simulink model "Marine_LocoMotive_UAV"  (R2018a)
settings: Solver=ode4  StartTime=0.0  StopTime=80  FixedStep=T  RelTol=1e-3
values from neighbouring files (symbols this model uses):
  a_11 = 0.05*m_b    (= 0.625)    [Marine_LocoMotive_UAV.m]
  a_33 = m_b    (= 12.5)    [Marine_LocoMotive_UAV.m]
  A_w = 1*1.5/2    (= 0.75)    [Marine_LocoMotive_UAV.m]
  A_w2 = 1*0.27/2    (= 0.135)    [Marine_LocoMotive_UAV.m]
  Ac = 0.0331    [Marine_LocoMotive_UAV.m]
  alpha_bar = pi/4    (= 0.785398163397)    [Marine_LocoMotive_UAV.m]
  Am = sysd.denominator{1}    [Marine_LocoMotive_UAV.m]
  Am1_LPF = sysd.denominator{1}    [Marine_LocoMotive_UAV.m]
  Am2_LPF = sysd.denominator{1}    [Marine_LocoMotive_UAV.m]
  Am_asw_LPF = sysd.denominator{1}    [Marine_LocoMotive_UAV.m]
  Am_coup_LPF = sysd.denominator{1}    [Marine_LocoMotive_UAV.m]
  Am_rdeL_LPF = sysd.denominator{1}    [Marine_LocoMotive_UAV.m]
  Am_reL_LPF = sysd.denominator{1}    [Marine_LocoMotive_UAV.m]
  Am_rref20_LPF = sysd.denominator{1}    [Marine_LocoMotive_UAV.m]
  Am_rref_LPF = sysd.denominator{1}    [Marine_LocoMotive_UAV.m]
  AmAlpha_LPF = sysd.denominator{1}    [Marine_LocoMotive_UAV.m]
  Amp_sf = 3    [Marine_LocoMotive_UAV.m]
  AmV_LPF = sysd.denominator{1}    [Marine_LocoMotive_UAV.m]
  AmZ_LPF = sysd.denominator{1}    [Marine_LocoMotive_UAV.m]
  b_11 = 0    [Marine_LocoMotive_UAV.m]
  b_33 = 2*m_b*omega_h    (= 27.5578302946)    [Marine_LocoMotive_UAV.m]
  Bm = sysd.numerator{1}    [Marine_LocoMotive_UAV.m]
  Bm1_LPF = sysd.numerator{1}    [Marine_LocoMotive_UAV.m]
  Bm2_LPF = sysd.numerator{1}    [Marine_LocoMotive_UAV.m]
  Bm_asw_LPF = sysd.numerator{1}    [Marine_LocoMotive_UAV.m]
  Bm_coup_LPF = sysd.numerator{1}    [Marine_LocoMotive_UAV.m]
  Bm_rdeL_LPF = sysd.numerator{1}    [Marine_LocoMotive_UAV.m]
  Bm_reL_LPF = sysd.numerator{1}    [Marine_LocoMotive_UAV.m]
  Bm_rref20_LPF = sysd.numerator{1}    [Marine_LocoMotive_UAV.m]
  Bm_rref_LPF = sysd.numerator{1}    [Marine_LocoMotive_UAV.m]
  BmAlpha_LPF = sysd.numerator{1}    [Marine_LocoMotive_UAV.m]
  BmV_LPF = sysd.numerator{1}    [Marine_LocoMotive_UAV.m]
  BmZ_LPF = sysd.numerator{1}    [Marine_LocoMotive_UAV.m]
  C_S = [5;9]*10^-3    [Marine_LocoMotive_UAV.m]
  Cd_u = 0.2    [Marine_LocoMotive_UAV.m]
  D_x = b_11 + D_s(1)    [Marine_LocoMotive_UAV.m]
  D_z = b_33 + D_s(2)    [Marine_LocoMotive_UAV.m]
  dc_M_p = 6.7    [Marine_LocoMotive_UAV.m]
  Delta_h = (A_im/A_b-0.5)*h_b    (= -0.0625)    [Marine_LocoMotive_UAV.m]
  eps_V = 0.1    [Marine_LocoMotive_UAV.m]
  epsilon_1 = 5    [Marine_LocoMotive_UAV.m]
  epsilon_e_u1 = 0.05    [Marine_LocoMotive_UAV.m]
  epsilon_w = 0    [Marine_LocoMotive_UAV.m]
  epsilon_w2 = pi    (= 3.14159265359)    [Marine_LocoMotive_UAV.m]
  g = 9.81    [Marine_LocoMotive_UAV.m]
  gamma_d_p = (2*0.3/0.03*2*0.2*12/4)/10    (= 2.4)    [Marine_LocoMotive_UAV.m]
  H = 10    [Marine_LocoMotive_UAV.m]
  h_b = 0.25    [Marine_LocoMotive_UAV.m]
  J_b = m_b*h_b*l_b/12    (= 0.208333333333)    [Marine_LocoMotive_UAV.m]
  J_u = 0.03    [Marine_LocoMotive_UAV.m]
  K = 40    [Marine_LocoMotive_UAV.m]
  k3 = 24    [Marine_LocoMotive_UAV.m]
  k4 = 0.8    [Marine_LocoMotive_UAV.m]
  k_w = omega_w^2/g    (= 0.123862835563)    [Marine_LocoMotive_UAV.m]
  k_w2 = omega_w2^2/g    (= 0.447144836384)    [Marine_LocoMotive_UAV.m]
  kd_a = 5.6    [Marine_LocoMotive_UAV.m]
  kd_r = 19.5    [Marine_LocoMotive_UAV.m]
  kd_t = 10    [Marine_LocoMotive_UAV.m]
  kd_x = 5    [Marine_LocoMotive_UAV.m]
  kd_z = 2    [Marine_LocoMotive_UAV.m]
  ki_a = 1.6    [Marine_LocoMotive_UAV.m]
  ki_r = 9    [Marine_LocoMotive_UAV.m]
  ki_T = 12    [Marine_LocoMotive_UAV.m]
  ki_x = 1.2    [Marine_LocoMotive_UAV.m]
  ki_z = 1    [Marine_LocoMotive_UAV.m]
  kp_a = 9.6    [Marine_LocoMotive_UAV.m]
  kp_r = 45    [Marine_LocoMotive_UAV.m]
  kp_t = 20    [Marine_LocoMotive_UAV.m]
  kp_T = 25    [Marine_LocoMotive_UAV.m]
  kp_x = 7    [Marine_LocoMotive_UAV.m]
  kp_z = 3    [Marine_LocoMotive_UAV.m]
  L = 0.2    [Marine_LocoMotive_UAV.m]
  l_b = 0.8    [Marine_LocoMotive_UAV.m]
  Lc_0 = 7    [Marine_LocoMotive_UAV.m]
  LIMIT_CMD_PITCH = 45*pi/180    (= 0.785398163397)    [Marine_LocoMotive_UAV.m]
  LIMIT_uCMD_HEIGHT = 3.5*K    (= 140)    [Marine_LocoMotive_UAV.m]
  m_b = rho_w*Vol_b/4    (= 12.5)    [Marine_LocoMotive_UAV.m]
  m_u = 1.8    [Marine_LocoMotive_UAV.m]
  min_sf = 5    [Marine_LocoMotive_UAV.m]
  nu_w = 1.787*10^-6    (= 1.787e-06)    [Marine_LocoMotive_UAV.m]
  omega_w = 2*pi/T_w    (= 1.10231321179)    [Marine_LocoMotive_UAV.m]
  omega_w2 = 2*pi/T_w2    (= 2.09439510239)    [Marine_LocoMotive_UAV.m]
  r_0 = sqrt( (X0_b(1) - X0_u(1))^2 +(X0_b(2) - X0_u(2))^2 )    [Marine_LocoMotive_UAV.m]
  r_bar = Lc_0-0.3    (= 6.7)    [Marine_LocoMotive_UAV.m]
  r_min = (zu_bar-H)-0.2    [Marine_LocoMotive_UAV.m]
  rho_a = 1.225    [Marine_LocoMotive_UAV.m]
  rho_w = 1000    [Marine_LocoMotive_UAV.m]
  T = 1/500    (= 0.002)    [Marine_LocoMotive_UAV.m]
  T_init = 10    [Marine_LocoMotive_UAV.m]
  Theta0 = 0*atan2(V_bar*D_x*cos(alpha_bar_0),V_bar*D_x*sin(alpha_bar_0)+m_u*g*cos(alpha_bar_0))    [Marine_LocoMotive_UAV.m]
  u_s = w_dir*A_w^2*omega_w*k_w*exp(2*k_w*(-Delta_h/2))    [Marine_LocoMotive_UAV.m]
  u_s2 = w_dir2*A_w2^2*omega_w2*k_w2*exp(2*k_w2*(-Delta_h/2))    [Marine_LocoMotive_UAV.m]
  u_t = -1*0.5*1    (= -0.5)    [Marine_LocoMotive_UAV.m]
  u_w = 0*0.2    (= 0)    [Marine_LocoMotive_UAV.m]
  V0_b = [u_t+u_w+u_s+v_x_w, v_z_w]    [Marine_LocoMotive_UAV.m]
  V0_u = [0 0]    [Marine_LocoMotive_UAV.m]
  V_bar = 4    [Marine_LocoMotive_UAV.m]
  Vol_b = A_b*l_b    (= 0.05)    [Marine_LocoMotive_UAV.m]
  w_dir = 1    [Marine_LocoMotive_UAV.m]
  w_dir2 = 1    [Marine_LocoMotive_UAV.m]
  X0_b = [0,H-Delta_h]    [Marine_LocoMotive_UAV.m]
  X0_u = X0_b + [3 3]    [Marine_LocoMotive_UAV.m]
  zu_bar = X0_b(2) + Lc_0*sin(alpha_bar_0)    [Marine_LocoMotive_UAV.m]
undefined symbols (not defined in the file or in its folder): Am_HPF, Am_LPF, Am_LPF2, an1, an1_v, an2, an3, Bm_HPF, Bm_LPF, Bm_LPF2, bn1, bn1_v, bn2, bn3, DiscIntNeverNeededParam, F, Light, magnitude, MIL, OMEGA_FILTER_OUTER, R_b, Tc, Tg, Tn, Ts, Tsc, Tz, X_GPS_offset
libraries: simulink x50, simulink_extras x9, aerolibwind2 x2
(part 3 of 6)

== system Marine_LocoMotive_UAV/Sensors and Filters/Sensors ==
  note: Gyro noise destroys the estimation
  note: Acc noise does not affect estimation
  "q " : Inport
  Ab : Inport  Port=2
  Xe : Inport  Port=3
  Euler : Inport  Port=4
  " Sonar (10Hz) (true elevation instead real sonar signal)" : Subsystem
  Accelerometer (500Hz) : Subsystem  TreatAsAtomicUnit=on  SystemSampleTime=Ts
  "GPS (10Hz) " : Subsystem  TreatAsAtomicUnit=on  SystemSampleTime=Tg
  Gyro (500Hz) : Subsystem  TreatAsAtomicUnit=on  SystemSampleTime=Ts
  RT : RateTransition  OutPortSampleTime=Ts
  Rate Transition : RateTransition
  Rate Transition1 : RateTransition
  Rate Transition2 : RateTransition  Deterministic=off  InitialCondition=[X0_u Theta0 1 1]
  Z : Selector  InputPortWidth=5  IndexOptions=Index vector (dialog)  Indices=2  OutputSizes=1
  acc : Scope  Commented=on
  pqr : Scope  Commented=on
  rotation matrix R : Subsystem
  Acc : Outport
  GPS : Outport  Port=2
  " q" : Outport  Port=3
  Sonar : Outport  Port=4
  wires:
  Xe/1 -> "GPS (10Hz) "/1(Xe)
  Ab/1 -> RT/1
  "q "/1 -> Gyro (500Hz)/1(q)
  Euler/1 -> rotation matrix R/1(angle (rad)), "GPS (10Hz) "/2(Euler)
  Accelerometer (500Hz)/1(Acc) -> Rate Transition1/1
  Gyro (500Hz)/1(" q") -> Rate Transition/1
  Z/1 -> " Sonar (10Hz) (true elevation instead real sonar signal)"/1(sonar (m))
  " Sonar (10Hz) (true elevation instead real sonar signal)"/1(calib sonar (m)) -> Sonar/1
  Rate Transition/1 -> pqr/1, " q"/1
  Rate Transition1/1 -> acc/1, Acc/1
  RT/1 -> Accelerometer (500Hz)/1(Ab)
  rotation matrix R/1(R) -> "GPS (10Hz) "/3(DCM_b2e)
  Rate Transition2/1 -> Z/1, GPS/1
  "GPS (10Hz) "/1(GPS) -> Rate Transition2/1

== system Marine_LocoMotive_UAV/Sensors and Filters/Sterio camera + encoder ==
  note: the error in alpha should relate to the stereo camera accuracy and the radial distance:
      | alpha = atan( 2cm / 7 m) = 0.0029 rad.
  alpha : Inport
  alpha_dot : Inport  Port=2
  alpha_ddot : Inport  Port=3
  r : Inport  Port=4
  r_dot : Inport  Port=5
  r_ddot : Inport  Port=6
  Discrete Derivative{,1..3} (4 alike) : simulink/Discrete/Discrete Derivative  gainval=1.0  ICPrevScaledInput=0.0  OutMin=[]  OutMax=[]  OutDataType=fixdt(1, 16)  OutScaling=2^-10  DoSatur=off
  Gain1 : Gain  Gain=0.5
  Gain2 : Gain  Gain=0.3
  Gain4 : Gain
  Gain5 : Gain
  Gain6 : Gain  Gain=0.25
  Gain7 : Gain  Gain=0.5
  Low Pass Filter{1..9} (9 alike) : DiscreteTransferFcn  Numerator=Bm_LPF2  Denominator=Am_LPF2
  Low Pass Filter10 : DiscreteTransferFcn  Commented=on  Numerator=Bm_LPF2  Denominator=Am_LPF2
  Low Pass Filter11 : DiscreteTransferFcn  Commented=on  Numerator=Bm_LPF2  Denominator=Am_LPF2
  Rate Transition1 : RateTransition
  Rate Transition2 : RateTransition
  Sum{1..2,7..10} (6 alike) : Sum  Inputs=++|
  stereo cam noise (location in frame) : RandomNumber  Variance=1/100000  Seed=5684  SampleTime=Tsc
  sterio cam noise (range) : RandomNumber  Variance=1/1000  Seed=1142  SampleTime=Tsc
  alpha_est : Outport
  alpha_dot_est : Outport  Port=2
  r_est : Outport  Port=3
  r_dot_est : Outport  Port=4
  alpha_ddot_est : Outport  Port=5
  r_ddot_est : Outport  Port=6
  wires:
  Rate Transition2/1 -> Low Pass Filter3/1
  stereo cam noise (location in frame)/1 -> Rate Transition2/1
  Gain5/1 -> Sum8/1
  Sum10/1 -> r_dot_est/1
  Discrete Derivative/1 -> Low Pass Filter8/1
  alpha_dot/1 -> Sum9/2
  Gain4/1 -> Sum7/1
  Discrete Derivative1/1 -> Low Pass Filter7/1
  Sum7/1 -> alpha_est/1
  Sum8/1 -> r_est/1
  r/1 -> Sum8/2
  alpha/1 -> Sum7/2
  r_dot/1 -> Sum10/2
  Sum9/1 -> alpha_dot_est/1
  sterio cam noise (range)/1 -> Rate Transition1/1
  Rate Transition1/1 -> Low Pass Filter1/1
  Sum1/1 -> alpha_ddot_est/1
  Discrete Derivative2/1 -> Low Pass Filter6/1
  Gain6/1 -> Discrete Derivative2/1, Sum9/1
  Gain1/1 -> Sum1/1
  alpha_ddot/1 -> Sum1/2
  r_ddot/1 -> Sum2/2
  Discrete Derivative3/1 -> Low Pass Filter9/1
  Gain2/1 -> Sum2/1
  Sum2/1 -> r_ddot_est/1
  Gain7/1 -> Discrete Derivative3/1, Sum10/1
  Low Pass Filter2/1 -> Gain7/1
  Low Pass Filter4/1 -> Gain2/1
  Low Pass Filter5/1 -> Gain6/1
  Low Pass Filter6/1 -> Gain1/1
  Low Pass Filter7/1 -> Low Pass Filter5/1
  Low Pass Filter8/1 -> Low Pass Filter2/1
  Low Pass Filter9/1 -> Low Pass Filter4/1
  Low Pass Filter3/1 -> Gain4/1, Discrete Derivative1/1
  Low Pass Filter1/1 -> Gain5/1, Discrete Derivative/1

== system Marine_LocoMotive_UAV/Sensors and Filters/quadrotor position from relative buoy-UAV position ==
  X_u : Inport
  Xdot_u : Inport  Port=2
  Xddot_u : Inport  Port=3
  r : Inport  Port=4
  r_dot : Inport  Port=5
  r_ddot : Inport  Port=6
  alpha : Inport  Port=7
  alpha_dot : Inport  Port=8
  alpha_ddot : Inport  Port=9
  Demux : Demux  Outputs=2
  Gain1 : Gain  Gain=-1
  Gain2 : Gain  Gain=2
  Product1 : Product  Inputs=3
  Product{2,4..5,7..8} (5 alike) : Product
  Product3 : Product  Multiplication=Matrix(*)
  Product6 : Product  Multiplication=Matrix(*)
  Sum : Sum  Inputs=|+-
  Sum1 : Sum  Inputs=|+-
  Sum2 : Sum  Inputs=+-|
  Sum3 : Sum  Inputs=++|
  Sum4 : Sum  Inputs=+-|
  Trigonometric Function : Trigonometry  Operator=sincos
  Vector Concatenate{1..4} (4 alike) : Concatenate
  r1 : InportShadow  Port=4
  r_dot1 : InportShadow  Port=5
  "rotation matrix R " : Subsystem
  theta u{1..2,4,6} (4 alike) : Scope
  Xb : Outport
  Xdot_b : Outport  Port=2
  Xddot_b : Outport  Port=3
  wires:
  Trigonometric Function/2 -> Product5/1
  Trigonometric Function/1 -> Product4/1
  alpha/1 -> "rotation matrix R "/1(angle (rad)), Trigonometric Function/1  "alpha"
  Sum1/1 -> Vector Concatenate3/2
  Vector Concatenate3/1 -> theta u4/1, Xb/1
  Product5/1 -> Sum/2
  Demux/2 -> Sum1/1  "z_u"
  Product4/1 -> Sum1/2
  Sum/1 -> Vector Concatenate3/1
  X_u/1 -> Demux/1
  Demux/1 -> Sum/1  "x_u"
  Vector Concatenate2/1 -> Product3/2
  Sum4/1 -> Xdot_b/1, theta u6/1
  Product3/1 -> Sum4/2
  r/1 -> Product2/1, Product5/2, Product4/2
  r_dot/1 -> theta u1/1, Vector Concatenate2/1
  Product2/1 -> theta u2/1, Vector Concatenate2/2
  alpha_dot/1 -> Product2/2, Product7/1, Product1/2, Product1/1
  Xdot_u/1 -> Sum4/1
  Product6/1 -> Sum2/2
  Gain2/1 -> Vector Concatenate1/2
  "rotation matrix R "/1(R) -> Product6/1, Product3/1
  Product1/1 -> Gain1/1
  Sum3/1 -> Product6/2
  r1/1 -> Product8/1, Product1/3
  Product7/1 -> Gain2/1
  r_dot1/1 -> Product7/2
  Xddot_u/1 -> Sum2/1
  Vector Concatenate1/1 -> Sum3/2
  r_ddot/1 -> Vector Concatenate4/1
  Product8/1 -> Vector Concatenate4/2
  alpha_ddot/1 -> Product8/2
  Vector Concatenate4/1 -> Sum3/1
  Gain1/1 -> Vector Concatenate1/1
  Sum2/1 -> Xddot_b/1

== system Marine_LocoMotive_UAV/UAV controller/Coupling ==
  U1 : Inport
  U3 : Inport  Port=2
  Coupling : Subsystem
  sat : Subsystem
  u_1 : Outport
  theta_d : Outport  Port=2
  wires:
  Coupling/1(u1 (N)) -> u_1/1
  Coupling/2(phi_d (rad)) -> sat/1(u)
  U3/1 -> Coupling/2(U3)
  U1/1 -> Coupling/1(U1)
  sat/1(sat(u)) -> theta_d/1

== system Marine_LocoMotive_UAV/UAV controller/Coupling  ==
  u_T : Inport
  u_a : Inport  Port=2
  alpha : Inport  Port=3
  Add5 : Sum  Inputs=2
  Bias : Bias  Bias=-pi/2
  Product1 : Product
  Product3 : Product
  Saturation : Saturate  UpperLimit=LIMIT_uCMD_HEIGHT  LowerLimit=m_u*g*0.5
  Scope{,1..5} (6 alike) : Scope
  Sqrt : Sqrt  SaturateOnIntegerOverflow=on
  Subtract : Sum  Inputs=--
  Trigonometric Function1 : Trigonometry  Operator=atan2
  Vector Concatenate : Concatenate
  "sat " : Subsystem
  u1 : Outport
  theta_c : Outport  Port=2
  wires:
  Bias/1 -> Scope2/1, Subtract/1
  Product1/1 -> Add5/1, Scope/1
  Sqrt/1 -> Saturation/1
  Subtract/1 -> "sat "/1(u)
  Trigonometric Function1/1 -> Scope4/1, Subtract/2
  Product3/1 -> Scope1/1, Add5/2
  Add5/1 -> Sqrt/1
  alpha/1 -> Bias/1
  Saturation/1 -> u1/1
  "sat "/1(sat(u)) -> Scope3/1, theta_c/1
  u_a/1 -> Vector Concatenate/1, Trigonometric Function1/1, Product3/1, Product3/2
  u_T/1 -> Product1/2, Product1/1, Vector Concatenate/2, Trigonometric Function1/2
  Vector Concatenate/1 -> Scope5/1

== system Marine_LocoMotive_UAV/UAV controller/Enabled Subsystem1 ==
  u : Inport
  reset : Inport  Port=2
  u0 : Inport  Port=3
  Enable : EnablePort
  Logical Operator : Logic  Operator=NOT  AllPortsSameDT=off  OutDataTypeStr=boolean
  Low Pass Filter5 : DiscreteTransferFcn  Numerator=Bm_rdeL_LPF  Denominator=Am_rdeL_LPF  InitialStatesSource=Input port  ExternalReset=Level
      settings: InputPortMap=u0,r7,p5
  Mux2 : Mux  Inputs=2
  adjustment for this specific transfer function : Gain  Gain=84.6505602
  r_dot filt : Scope
  r_dot filt1 : Scope
  y : Outport
  wires:
  u/1 -> Mux2/2, Low Pass Filter5/1
  Low Pass Filter5/1 -> Mux2/1, y/1
  Logical Operator/1 -> r_dot filt1/1, Low Pass Filter5/2
  u0/1 -> adjustment for this specific transfer function/1
  Mux2/1 -> r_dot filt/1
  adjustment for this specific transfer function/1 -> Low Pass Filter5/3
  reset/1 -> Logical Operator/1

== system Marine_LocoMotive_UAV/UAV controller/V controller ==
  V_bar : Inport
  V : Inport  Port=2
  Discrete Derivative1 : simulink/Discrete/Discrete Derivative  gainval=1.0  ICPrevScaledInput=0.0  OutMin=[]  OutMax=[]  OutDataType=fixdt(1, 16)  OutScaling=2^-10  DoSatur=off
  Discrete Derivative6 : simulink/Discrete/Discrete Derivative  gainval=1.0  ICPrevScaledInput=0.0  OutMin=[]  OutMax=[]  OutDataType=fixdt(1, 16)  OutScaling=2^-10  DoSatur=off
  Discrete-Time Integrator : DiscreteIntegrator  SampleTime=-1  LimitOutput=on  UpperSaturationLimit=300  LowerSaturationLimit=-200  ICPrevOutput=DiscIntNeverNeededParam  ICPrevScaledInput=DiscIntNeverNeededParam
  Gain : Gain  Gain=ki_x
  IC : InitialCondition  Value=0
  IC1 : InitialCondition  Value=0
  IC2 : InitialCondition  Value=0
  K1 : Gain  Gain=kp_x
  K2 : Gain  Gain=kd_x
  K3 : Gain
  K4 : Gain
  Mux : Mux  Inputs=2
  Mux1 : Mux  Inputs=2
  Product : Product
  Saturation1 : Saturate  UpperLimit=50  LowerLimit=-20
  Scope{1..6} (6 alike) : Scope
  Step : Step  Time=3*T  SampleTime=0
  Sum : Sum  Inputs=|+-
  Sum1 : Sum  Inputs=|+-
  Sum4 : Sum  Inputs=---
  U1 (m/s^2) : Outport
  wires:
  Sum1/1 -> Product/1  "ev"
  Sum/1 -> Discrete-Time Integrator/1, K1/1  "ex"
  V_bar/1 -> Mux/2, Sum/2, Discrete Derivative6/1
  Sum4/1 -> Saturation1/1
  K1/1 -> K4/1
  K2/1 -> K3/1
  Discrete-Time Integrator/1 -> Gain/1
  Gain/1 -> Scope3/1, Sum4/3
  Saturation1/1 -> Scope4/1, U1 (m/s^2)/1
  Mux/1 -> Scope1/1
  Discrete Derivative1/1 -> IC1/1
  Mux1/1 -> Scope2/1
  Discrete Derivative6/1 -> IC2/1
  IC/1 -> Discrete Derivative1/1, Mux/1, Sum/1
  V/1 -> IC/1
  IC1/1 -> Sum1/1, Mux1/1
  IC2/1 -> Mux1/2, Sum1/2
  K3/1 -> Scope5/1, Sum4/2
  K4/1 -> Scope6/1, Sum4/1
  Product/1 -> K2/1
  Step/1 -> Product/2

== system Marine_LocoMotive_UAV/UAV controller/Z controller ==
  z_bar : Inport
  z_u : Inport  Port=2
  Constant : Constant  Value=g
  Discrete Derivative1 : simulink/Discrete/Discrete Derivative  gainval=1.0  ICPrevScaledInput=0.0  OutMin=[]  OutMax=[]  OutDataType=fixdt(1, 16)  OutScaling=2^-10  DoSatur=off
  Discrete Derivative6 : simulink/Discrete/Discrete Derivative  gainval=1.0  ICPrevScaledInput=0.0  OutMin=[]  OutMax=[]  OutDataType=fixdt(1, 16)  OutScaling=2^-10  DoSatur=off
  Discrete-Time Integrator : DiscreteIntegrator  SampleTime=-1  LimitOutput=on  UpperSaturationLimit=100  LowerSaturationLimit=-100  ICPrevOutput=DiscIntNeverNeededParam  ICPrevScaledInput=DiscIntNeverNeededParam
  Divide : Product  Inputs=*/
  Gain : Gain  Gain=ki_z
  IC : InitialCondition  Value=0
  IC1 : InitialCondition  Value=0
  K1 : Gain  Gain=kp_z
  K2 : Gain  Gain=kd_z
  K3 : Gain
  Mux : Mux  Inputs=2
  Mux1 : Mux  Inputs=2
  Saturation1 : Saturate  UpperLimit=inf  LowerLimit=g/2
  Scope{1..6} (6 alike) : Scope
  Sum : Sum  Inputs=|+-
  Sum1 : Sum  Inputs=|+-
  Sum2 : Sum  Inputs=|++
  Sum4 : Sum  Inputs=---
  Trigonometric Function : Trigonometry  Operator=cos
  U3 (m/s^2) : Outport
  wires:
  Gain/1 -> Scope3/1, Sum4/3
  Discrete-Time Integrator/1 -> Gain/1
  K2/1 -> Scope5/1, Sum4/2
  K1/1 -> K3/1
  Sum4/1 -> Sum2/1
  Discrete Derivative1/1 -> IC/1
  Discrete Derivative6/1 -> IC1/1
  z_u/1 -> Discrete Derivative1/1, Mux/1, Sum/1
  Sum/1 -> K1/1, Discrete-Time Integrator/1  "ex"
  Sum1/1 -> K2/1  "ev"
  z_bar/1 -> Mux/2, Sum/2, Discrete Derivative6/1
  Mux/1 -> Scope1/1
  Mux1/1 -> Scope2/1
  Saturation1/1 -> U3 (m/s^2)/1, Scope4/1
  IC/1 -> Mux1/1, Sum1/1
  IC1/1 -> Mux1/2, Sum1/2
  K3/1 -> Scope6/1, Sum4/1
  [theta_u] -> Trigonometric Function/1
  Trigonometric Function/1 -> Divide/2
  Sum2/1 -> Saturation1/1
  Constant/1 -> Divide/1
  Divide/1 -> Sum2/2

== system Marine_LocoMotive_UAV/UAV controller/cond1 ==
  r : Inport
  r_dot : Inport  Port=2
  coupled : Inport  Port=3
  Constant : Constant  Value=Lc_0
  Constant2 : Constant  Value=T
  MATLAB Function : MATLAB Function  TreatAsAtomicUnit=on
  r_dot filt2 : Scope
  key : Outport
  wires:
  r/1 -> MATLAB Function/1(r)
  Constant/1 -> MATLAB Function/4(Lc)
  Constant2/1 -> MATLAB Function/5(dt)
  MATLAB Function/1(y) -> key/1
  r_dot/1 -> MATLAB Function/2(r_dot)
  coupled/1 -> MATLAB Function/3(coupled)
  MATLAB Function/2(t) -> r_dot filt2/1

== system Marine_LocoMotive_UAV/UAV controller/pitch control ==
  theta_d : Inport
  theta_q : Inport  Port=2
  omega_q : Inport  Port=3
  Constant : Constant  Value=J_u
  Discrete Transfer Fcn : DiscreteTransferFcn  Numerator=Bm1_LPF  Denominator=Am1_LPF
  Discrete Transfer Fcn1 : DiscreteTransferFcn  Numerator=Bm2_LPF  Denominator=Am2_LPF
  Discrete Derivative3 : simulink/Discrete/Discrete Derivative  gainval=1.0  ICPrevScaledInput=Theta0/T  OutMin=[]  OutMax=[]  OutDataType=fixdt(1, 16)  OutScaling=2^-10  DoSatur=off
  Discrete Derivative4 : simulink/Discrete/Discrete Derivative  gainval=1.0  ICPrevScaledInput=0.0  OutMin=[]  OutMax=[]  OutDataType=fixdt(1, 16)  OutScaling=2^-10  DoSatur=off
  Discrete Derivative6 : simulink/Discrete/Discrete Derivative  gainval=1.0  ICPrevScaledInput=Theta0/T  OutMin=[]  OutMax=[]  OutDataType=fixdt(1, 16)  OutScaling=2^-10  DoSatur=off
  Discrete-Time Integrator : DiscreteIntegrator  SampleTime=-1  LimitOutput=on  UpperSaturationLimit=dc_M_p  LowerSaturationLimit=-dc_M_p  ICPrevOutput=DiscIntNeverNeededParam  ICPrevScaledInput=DiscIntNeverNeededParam
  Gain : Gain  Gain=gamma_d_p
  IC : InitialCondition  Value=0
  IC2 : InitialCondition  Value=0
  Integrator : Integrator  Commented=on  LimitOutput=on  UpperSaturationLimit=dc_M_p  LowerSaturationLimit=-dc_M_p
  K1 : Gain  Gain=kp_t
  K2 : Gain  Gain=kd_t
  K3 : Gain  Gain=1+k3*k4
  K4 : Gain  Gain=k3+k4
  K5 : Gain
  K6 : Gain
  Mux : Mux  Inputs=2
  Mux1 : Mux  Inputs=3
  Mux2 : Mux  Inputs=2
  Product1 : Product
  Saturation : Saturate  UpperLimit=[5]  LowerLimit=[-5]
  Saturation - Limit Height Controller1 : Saturate  UpperLimit=K*L*1.41/4  LowerLimit=-K*L*1.41/4
  Saturation - Limit Height Controller2 : Saturate  UpperLimit=15  LowerLimit=-15
  Sum : Sum  Inputs=|+-
  Sum1 : Sum  Inputs=|+-
  Sum4 : Sum  Inputs=--+-
  T2 {,1..9} (10 alike) : Scope
  theta_d1 : InportShadow
  M1 (N.m) : Outport
  wires:
  Product1/1 -> Saturation - Limit Height Controller1/1
  Saturation - Limit Height Controller1/1 -> "T2 "/1, M1 (N.m)/1
  Sum1/1 -> K2/1  "ev"
  Sum4/1 -> Product1/1
  Discrete Derivative6/1 -> IC/1
  Discrete Derivative3/1 -> IC2/1
  Discrete Transfer Fcn1/1 -> Mux2/1, Saturation/1
  Sum/1 -> K1/1, Discrete-Time Integrator/1  "ex"
  K1/1 -> T2 7/1, Sum4/1
  K2/1 -> K6/1
  Discrete-Time Integrator/1 -> Gain/1
  Gain/1 -> K5/1, T2 5/1
  Constant/1 -> Product1/2
  Mux/1 -> T2 1/1
  theta_q/1 -> Mux/1, Sum/1
  omega_q/1 -> Mux1/1, Sum1/1
  Mux1/1 -> T2 2/1
  Discrete Transfer Fcn/1 -> Mux1/2, Sum1/2  "ex"
  Discrete Derivative4/1 -> Mux2/2, Discrete Transfer Fcn1/1, T2 3/1
  theta_d/1 -> Mux/2, Sum/2, Discrete Derivative6/1
  Saturation/1 -> T2 8/1, Sum4/3
  IC/1 -> Mux1/3, Discrete Transfer Fcn/1
  theta_d1/1 -> Discrete Derivative3/1
  IC2/1 -> Discrete Derivative4/1
  K5/1 -> Sum4/4
  Mux2/1 -> T2 4/1
  K6/1 -> T2 6/1, Sum4/2

== system Marine_LocoMotive_UAV/UAV controller/rdot 0 ==
  X : Inport
  Trigger : TriggerPort  VariantControl=Variant
  Xu_init : Outport
  wires:
  X/1 -> Xu_init/1

== system Marine_LocoMotive_UAV/UAV controller/switch controllers ==
  radial position : Inport
  buoy velocity : Inport  Port=2
  coupled : Inport  Port=3
  active : Inport  Port=4
  r : Inport  Port=5
  Abs1 : Abs  Commented=on
  Compare To Constant : simulink/Logic and Bit Operations/Compare To Constant  relop=>=  const=Lc_0-0.1  OutDataTypeStr=boolean
  Compare To Constant1 : simulink/Logic and Bit Operations/Compare To Constant  Commented=on  relop=<=  const=0.3  OutDataTypeStr=boolean
  Logical Operator1 : Logic  AllPortsSameDT=off  OutDataTypeStr=boolean
  Logical Operator2 : Logic  Operator=OR  AllPortsSameDT=off  OutDataTypeStr=boolean
  Mux1 : Mux  Inputs=2
  Mux2 : Mux  Inputs=2
  Smooth channel switching : Subsystem  Commented=on
  Switch : Switch  Criteria=u2 > Threshold
  smooth switch : Subsystem
  u_T1 : Scope
  u_T2 : Scope
  u_T3 : Scope
  u_T : Outport
  wires:
  buoy velocity/1 -> smooth switch/2(u 2), Switch/1, Mux2/2
  Logical Operator1/1 -> u_T2/1, smooth switch/3(switch), Switch/2
  coupled/1 -> Logical Operator2/2
  radial position/1 -> smooth switch/1(u 1), Switch/3, Mux2/1
  Switch/1 -> Mux1/1
  Mux2/1 -> u_T1/1
  active/1 -> Logical Operator1/2
  Logical Operator2/1 -> Logical Operator1/1
  r/1 -> Compare To Constant/1
  Compare To Constant/1 -> Logical Operator2/1
  Abs1/1 -> Compare To Constant1/1
  Mux1/1 -> u_T3/1
  smooth switch/1(y) -> u_T/1, Mux1/2

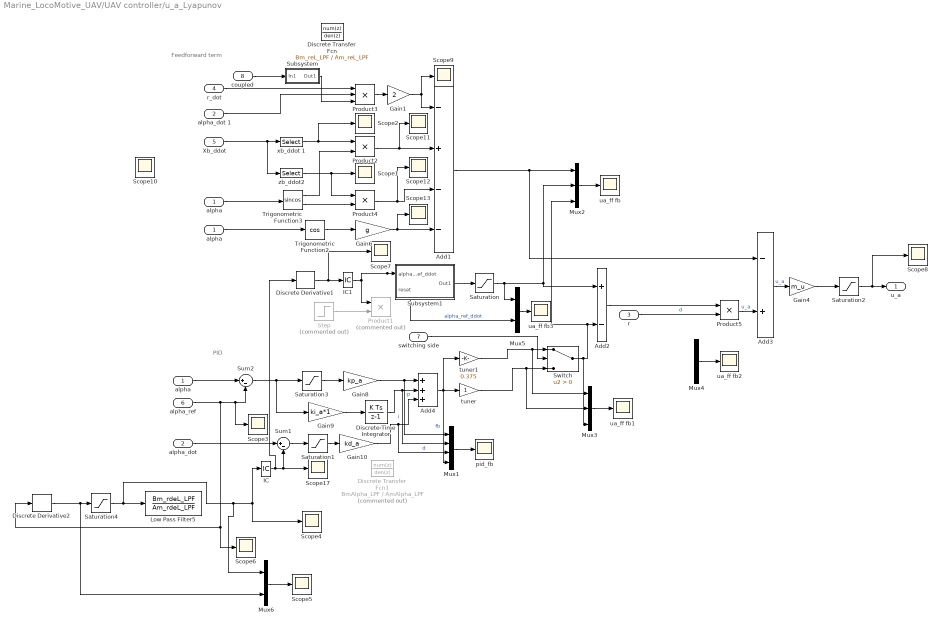
== system Marine_LocoMotive_UAV/UAV controller/u_a_Lyapunov ==
  note: Feedforward term
  note: PID
  alpha : Inport
  "alpha_dot " : Inport  Port=2
  r : Inport  Port=3
  r_dot : Inport  Port=4
  Xb_ddot : Inport  Port=5
  alpha_ref : Inport  Port=6
  switching side : Inport  Port=7
  coupled : Inport  Port=8
  " alpha" : InportShadow
  Add1 : Sum  Inputs=-+--
  Add2 : Sum  Inputs=+-
  Add3 : Sum  Inputs=-+
  Add4 : Sum  Inputs=3
  Discrete Transfer Fcn : DiscreteTransferFcn  Numerator=Bm_reL_LPF  Denominator=Am_reL_LPF
  Discrete Transfer Fcn1 : DiscreteTransferFcn  Commented=on  Numerator=BmAlpha_LPF  Denominator=AmAlpha_LPF
  Discrete Derivative1 : simulink/Discrete/Discrete Derivative  gainval=1.0  ICPrevScaledInput=alpha_bar  OutMin=[]  OutMax=[]  OutDataType=fixdt(1, 16)  OutScaling=2^-10  DoSatur=off
  Discrete Derivative2 : simulink/Discrete/Discrete Derivative  gainval=1.0  ICPrevScaledInput=alpha_bar/T  OutMin=[]  OutMax=[]  OutDataType=fixdt(1, 16)  OutScaling=2^-10  DoSatur=off
  Discrete-Time Integrator : DiscreteIntegrator  SampleTime=-1  LimitOutput=on  UpperSaturationLimit=1  LowerSaturationLimit=-1  ICPrevOutput=DiscIntNeverNeededParam  ICPrevScaledInput=DiscIntNeverNeededParam
  Gain1 : Gain  Gain=2
  Gain10 : Gain  Gain=kd_a
  Gain4 : Gain  Gain=m_u
  Gain6 : Gain  Gain=g
  Gain8 : Gain  Gain=kp_a
  Gain9 : Gain  Gain=ki_a*1
  IC : InitialCondition  Value=0
  IC1 : InitialCondition  Value=0
  Low Pass Filter5 : DiscreteTransferFcn  Numerator=Bm_rdeL_LPF  Denominator=Am_rdeL_LPF
  Mux1 : Mux
  Mux2 : Mux  Inputs=3
  Mux3 : Mux  Inputs=3
  Mux4 : Mux  Inputs=3
  Mux5 : Mux  Inputs=2
  Mux6 : Mux  Inputs=2
  Product1 : Product  Commented=on
  Product2 : Product
  Product3 : Product  Inputs=3
  Product4 : Product
  Product5 : Product
  Saturation : Saturate  UpperLimit=2  LowerLimit=-2
  Saturation1 : Saturate  UpperLimit=7  LowerLimit=-7
  Saturation2 : Saturate  UpperLimit=45  LowerLimit=-45
  Saturation3 : Saturate  UpperLimit=7*3.14/180  LowerLimit=-7*3.14/180
  Saturation4 : Saturate  UpperLimit=1  LowerLimit=-1
  Scope{1..13,17} (14 alike) : Scope
  Step : Step  Commented=on  Time=2*T  SampleTime=0
  Subsystem : Subsystem
  Subsystem1 : Subsystem
  Sum1 : Sum  Inputs=|+-
  Sum2 : Sum  Inputs=|+-
  Switch : Switch  Criteria=u2 > Threshold
  Trigonometric Function2 : Trigonometry  Operator=cos
  Trigonometric Function3 : Trigonometry  Operator=sincos
  "alpha " : InportShadow
  alpha_dot 1 : InportShadow  Port=2
  pid_fb : Scope
  tuner : Gain
  tuner1 : Gain  Gain=0.375
  ua_ff fb{,1..3} (4 alike) : Scope
  xb_ddot 1 : Selector  InputPortWidth=2  IndexOptions=Index vector (dialog)  Indices=1  OutputSizes=1
  zb_ddot2 : Selector  InputPortWidth=2  IndexOptions=Index vector (dialog)  Indices=2  OutputSizes=1
  u_a : Outport
  wires:
  Mux2/1 -> ua_ff fb/1
  Add1/1 -> Add3/1, Mux2/1
  Mux1/1 -> pid_fb/1
  alpha/1 -> Trigonometric Function2/1
  "alpha "/1 -> Trigonometric Function3/1
  " alpha"/1 -> Sum2/1
  Trigonometric Function3/2 -> Product4/2
  Discrete-Time Integrator/1 -> Add4/2, Mux1/2  "i"
  Trigonometric Function2/1 -> Gain6/1
  Trigonometric Function3/1 -> Product2/2
  Product2/1 -> Scope11/1, Add1/2
  Gain9/1 -> Discrete-Time Integrator/1
  xb_ddot 1/1 -> Product2/1, Scope2/1
  Gain10/1 -> Add4/3, Mux1/3  "d"
  Xb_ddot/1 -> xb_ddot 1/1, zb_ddot2/1
  Gain8/1 -> Add4/1, Mux1/1  "p"
  zb_ddot2/1 -> Product4/1, Scope1/1
  Switch/1 -> Mux3/3, Mux2/3, Add2/2
  Add3/1 -> Gain4/1  "u_a"
  "alpha_dot "/1 -> Sum1/1
  Add4/1 -> tuner/1, tuner1/1, Mux1/4  "fb"
  Sum1/1 -> Saturation1/1
  Sum2/1 -> Saturation3/1, Gain9/1
  Discrete Derivative2/1 -> Mux6/2, Saturation4/1
  Gain6/1 -> Scope13/1, Add1/4
  Product4/1 -> Scope12/1, Add1/3
  Discrete Derivative1/1 -> Scope7/1, IC1/1
  IC1/1 -> Saturation/1, Mux5/2, Subsystem1/1(alpha_ref_ddot), Product1/1  "alpha_ref_ddot"
  alpha_ref/1 -> Scope6/1, Discrete Derivative2/1, Scope3/1, Sum2/2
  Step/1 -> Product1/2
  IC/1 -> Discrete Derivative1/1, Sum1/2, Scope17/1
  alpha_dot 1/1 -> Product3/2
  Product3/1 -> Gain1/1
  Gain1/1 -> Scope9/1, Add1/1
  Add2/1 -> Product5/1
  Product5/1 -> Add3/2  "u_a"
  Gain4/1 -> Saturation2/1
  Saturation1/1 -> Gain10/1
  Saturation2/1 -> Scope8/1, u_a/1
  Saturation3/1 -> Gain8/1
  switching side/1 -> Switch/2
  tuner1/1 -> Mux3/1, Switch/1
  tuner/1 -> Mux3/2, Switch/3
  Mux3/1 -> ua_ff fb1/1
  r/1 -> Product5/2  "d"
  Mux4/1 -> ua_ff fb2/1
  r_dot/1 -> Product3/1
  Subsystem/1(Out1) -> Product3/3
  coupled/1 -> Subsystem/1(In1)
  Mux5/1 -> ua_ff fb3/1
  Saturation4/1 -> Mux6/1, IC/1, Scope4/1, Low Pass Filter5/1
  Mux6/1 -> Scope5/1
  Saturation/1 -> Mux5/1, Mux2/2, Add2/1

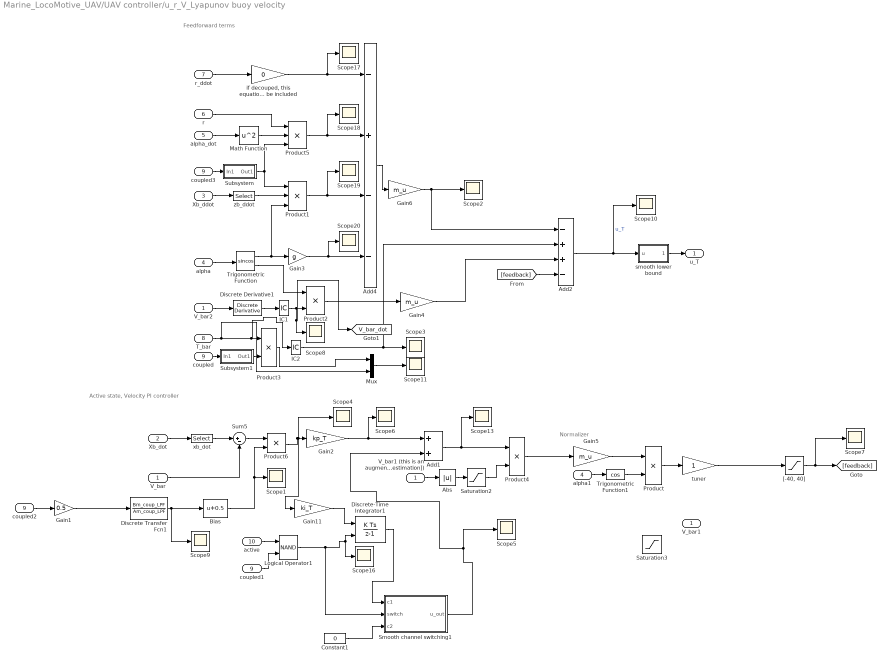
== system Marine_LocoMotive_UAV/UAV controller/u_r_V_Lyapunov buoy velocity ==
  note: Normalizer
  note: Feedforward terms
  note: Active state, Velocity PI controller
  V_bar : Inport
  Xb_dot : Inport  Port=2
  Xb_ddot : Inport  Port=3
  alpha : Inport  Port=4
  alpha_dot : Inport  Port=5
  r : Inport  Port=6
  r_ddot : Inport  Port=7
  T_bar : Inport  Port=8
  coupled : Inport  Port=9
  active : Inport  Port=10
  Abs : Abs
  Add1 : Sum
  Add2 : Sum  Inputs=-++-
  Add4 : Sum  Inputs=-+--
  Bias : Bias  Bias=0.5
  Constant1 : Constant  Value=0
  Discrete Transfer Fcn1 : DiscreteTransferFcn  Numerator=Bm_coup_LPF  Denominator=Am_coup_LPF
  Discrete Derivative1 : simulink/Discrete/Discrete Derivative  gainval=1.0  ICPrevScaledInput=V_bar/T  OutMin=[]  OutMax=[]  OutDataType=fixdt(1, 16)  OutScaling=2^-10  DoSatur=off
  Discrete-Time Integrator1 : DiscreteIntegrator  ExternalReset=level  SampleTime=-1  LimitOutput=on  UpperSaturationLimit=10  LowerSaturationLimit=-10  ICPrevOutput=DiscIntNeverNeededParam  ICPrevScaledInput=DiscIntNeverNeededParam
  Gain1 : Gain  Gain=0.5
  Gain11 : Gain  Gain=ki_T
  Gain2 : Gain  Gain=kp_T
  Gain3 : Gain  Gain=g
  Gain4 : Gain  Gain=m_u
  Gain5 : Gain  Gain=m_u
  Gain6 : Gain  Gain=m_u
  IC1 : InitialCondition  Value=0
  IC2 : InitialCondition  Value=0
  Logical Operator1 : Logic  Operator=NAND  AllPortsSameDT=off  OutDataTypeStr=boolean
  Math Function : Math  Operator=square  SaturateOnIntegerOverflow=on
  Mux : Mux  Inputs=2
  Product{,2..4,6} (5 alike) : Product
  Product1 : Product  Inputs=3
  Product5 : Product  Inputs=3
  Saturation2 : Saturate  UpperLimit=5  LowerLimit=1
  Saturation3 : Saturate  UpperLimit=5  LowerLimit=1
  Scope{1..11,13,16..20} (17 alike) : Scope
  Smooth channel switching1 : Subsystem
  Subsystem : Subsystem
  Subsystem1 : Subsystem
  Sum5 : Sum  Inputs=|+-
  Trigonometric Function : Trigonometry  Operator=sincos
  Trigonometric Function1 : Trigonometry  Operator=cos
  V_bar1 : InportShadow
  V_bar1 (this is an augmentation to the nominal controller for better drag compensation [error in tension estimation]) : InportShadow
  V_bar2 : InportShadow
  "[-40, 40]" : Saturate  UpperLimit=40  LowerLimit=-40
  alpha1 : InportShadow  Port=4
  coupled1 : InportShadow  Port=9
  coupled2 : InportShadow  Port=9
  coupled3 : InportShadow  Port=9
  "if decouped, this equation is not valid so r_ddot should not be included" : Gain  Gain=0
  smooth lower bound : Subsystem
  tuner : Gain
  xb_dot : Selector  InputPortWidth=2  IndexOptions=Index vector (dialog)  Indices=1  OutputSizes=1
  zb_ddot : Selector  InputPortWidth=2  IndexOptions=Index vector (dialog)  Indices=2  OutputSizes=1
  u_T : Outport
  tag scope: V_bar_dot=global
  wires:
  Gain5/1 -> Product/1
  smooth lower bound/1(sat(u)) -> u_T/1
  Add2/1 -> smooth lower bound/1(u), Scope10/1  "u_T"
  Xb_dot/1 -> xb_dot/1
  Discrete Derivative1/1 -> IC1/1
  Trigonometric Function/1 -> Product1/3, Gain3/1
  alpha/1 -> Trigonometric Function/1
  V_bar/1 -> Sum5/2
  Gain2/1 -> Add1/1, Scope6/1
  Product6/1 -> Gain2/1, Gain11/1, Scope4/1
  Smooth channel switching1/1(u_out) -> Scope5/1, Add1/2
  Product/1 -> tuner/1
  alpha1/1 -> Trigonometric Function1/1
  Xb_ddot/1 -> zb_ddot/1
  zb_ddot/1 -> Product1/2
  alpha_dot/1 -> Math Function/1
  Math Function/1 -> Product5/2
  Add4/1 -> Gain6/1
  Gain3/1 -> Scope20/1, Add4/4
  Product1/1 -> Scope19/1, Add4/3
  Product5/1 -> Scope18/1, Add4/2
  Gain6/1 -> Add2/1, Scope2/1
  IC1/1 -> Product2/2, [V_bar_dot], Scope8/1
  Product2/1 -> Gain4/1
  tuner/1 -> "[-40, 40]"/1
  V_bar2/1 -> Discrete Derivative1/1
  V_bar1 (this is an augmentation to the nominal controller for better drag compensation [error in tension estimation])/1 -> Abs/1
  Trigonometric Function/2 -> Product2/1
  Trigonometric Function1/1 -> Product/2
  Add1/1 -> Product4/1, Scope13/1
  [feedback] -> Add2/4
  Gain11/1 -> Discrete-Time Integrator1/1
  Saturation2/1 -> Product4/2
  IC2/1 -> Add2/2, Scope3/1
  r/1 -> Product5/1
  T_bar/1 -> Mux/2, IC2/1, Product3/1
  coupled/1 -> Subsystem1/1(In1)
  Gain4/1 -> Add2/3
  r_ddot/1 -> "if decouped, this equation is not valid so r_ddot should not be included"/1
  "if decouped, this equation is not valid so r_ddot should not be included"/1 -> Scope17/1, Add4/1
  xb_dot/1 -> Sum5/1
  coupled3/1 -> Subsystem/1(In1)
  active/1 -> Logical Operator1/1
  coupled1/1 -> Logical Operator1/2
  "[-40, 40]"/1 -> [feedback], Scope7/1
  Sum5/1 -> Product6/1
  Discrete Transfer Fcn1/1 -> Bias/1, Scope9/1
  Gain1/1 -> Discrete Transfer Fcn1/1
  coupled2/1 -> Gain1/1
  Bias/1 -> Product6/2, Scope1/1
  Product4/1 -> Gain5/1
  Abs/1 -> Saturation2/1
  Logical Operator1/1 -> Smooth channel switching1/2(switch), Scope16/1, Discrete-Time Integrator1/2
  Constant1/1 -> Smooth channel switching1/3(c2)
  Discrete-Time Integrator1/1 -> Smooth channel switching1/1(c1)
  Subsystem/1(Out1) -> Product5/3, Product1/1
  Subsystem1/1(Out1) -> Product3/2
  Product3/1 -> Mux/1
  Mux/1 -> Scope11/1

== system Marine_LocoMotive_UAV/UAV controller/u_r_p_Lyapunov radial position ==
  note: Feedforward terms
  note: Inactive state, position PID controller
  "r_bar " : Inport
  r : Inport  Port=2
  r_dot : Inport  Port=3
  alpha : Inport  Port=4
  alpha_dot : Inport  Port=5
  Xb_ddot : Inport  Port=6
  coupled : Inport  Port=7
  active : Inport  Port=8
  Add2 : Sum  Inputs=-+-
  Add3 : Sum  Inputs=3
  Add4 : Sum  Inputs=+---
  Discrete Derivative1 : simulink/Discrete/Discrete Derivative  gainval=1.0  ICPrevScaledInput=V_bar/T  OutMin=[]  OutMax=[]  OutDataType=fixdt(1, 16)  OutScaling=2^-10  DoSatur=off
  Discrete Derivative2 : simulink/Discrete/Discrete Derivative  gainval=1.0  ICPrevScaledInput=r_0/T  OutMin=[]  OutMax=[]  OutDataType=fixdt(1, 16)  OutScaling=2^-10  DoSatur=off
  Discrete-Time Integrator2 : DiscreteIntegrator  ExternalReset=level  SampleTime=-1  LimitOutput=on  UpperSaturationLimit=10  LowerSaturationLimit=-10  ICPrevOutput=DiscIntNeverNeededParam  ICPrevScaledInput=DiscIntNeverNeededParam
  Enabled Subsystem : Subsystem  TreatAsAtomicUnit=on
  Gain1 : Gain  Gain=ki_r
  Gain10 : Gain  Gain=kd_r
  Gain2 : Gain  Gain=m_u
  Gain3 : Gain  Gain=g
  Gain7 : Gain  Gain=kp_r
  IC1 : InitialCondition  Value=0
  Logical Operator1 : Logic  AllPortsSameDT=off  OutDataTypeStr=boolean
  Math Function : Math  Operator=square  SaturateOnIntegerOverflow=on
  Mux : Mux  Inputs=2
  Product1 : Product
  Product5 : Product
  Product7 : Product
  Scope{1..4,7..11,14..15,17..20} (15 alike) : Scope
  Sum1 : Sum  Inputs=|+-
  Sum3 : Sum  Inputs=-+|
  Trigonometric Function : Trigonometry  Operator=sincos
  cond : Subsystem
  "r  " : InportShadow  Port=2
  "r_bar  " : InportShadow
  tuner : Gain
  xb_ddot : Selector  InputPortWidth=2  IndexOptions=Index vector (dialog)  Indices=1  OutputSizes=1
  zb_ddot : Selector  InputPortWidth=2  IndexOptions=Index vector (dialog)  Indices=2  OutputSizes=1
  u_T : Outport
  wires:
  Add3/1 -> tuner/1
  Gain2/1 -> u_T/1, Scope1/1
  Add2/1 -> Gain2/1  "u_T"
  Discrete Derivative1/1 -> IC1/1
  Trigonometric Function/1 -> Gain3/1, Product1/2
  alpha/1 -> Trigonometric Function/1
  Xb_ddot/1 -> xb_ddot/1, zb_ddot/1
  zb_ddot/1 -> Product1/1
  alpha_dot/1 -> Math Function/1
  Math Function/1 -> Product5/2
  Gain3/1 -> Add4/4, Scope20/1
  Product1/1 -> Add4/3, Scope19/1
  Product5/1 -> Add4/1, Scope18/1
  Add4/1 -> Add2/1, Scope2/1  "Hr"
  tuner/1 -> [feedback], Scope7/1
  Discrete-Time Integrator2/1 -> Scope9/1, Add3/2
  "r  "/1 -> Sum1/1, Scope15/1
  Gain1/1 -> Discrete-Time Integrator2/1
  active/1 -> Logical Operator1/1
  Sum1/1 -> Gain7/1, Gain1/1, Scope14/1
  "r_bar  "/1 -> Sum1/2
  "r_bar "/1 -> Discrete Derivative2/1
  Trigonometric Function/2 -> Product7/2
  Sum3/1 -> Gain10/1
  Gain10/1 -> Add3/3, Scope10/1
  [feedback] -> Add2/3
  Gain7/1 -> Scope11/1, Add3/1
  Enabled Subsystem/1(y) -> Mux/2, Product5/1
  xb_ddot/1 -> Product7/1
  Product7/1 -> Add4/2, Scope17/1
  Discrete Derivative2/1 -> Sum3/1, Scope4/1, Discrete Derivative1/1
  r_dot/1 -> Sum3/2
  IC1/1 -> Add2/2, Scope8/1
  coupled/1 -> Logical Operator1/2
  Logical Operator1/1 -> Discrete-Time Integrator2/2
  r/1 -> Mux/1, Enabled Subsystem/1(u), cond/1(In1)
  cond/1(Out1) -> Enabled Subsystem/2(reset), Enabled Subsystem/Enable
  Mux/1 -> Scope3/1

== system Marine_LocoMotive_UAV/Wind model/magnitude ==
  In1 : Inport
  Math Function2 : Math  Operator=magnitude^2  SaturateOnIntegerOverflow=on
  Sqrt : Sqrt  SaturateOnIntegerOverflow=on
  Sum of Elements1 : Sum  Inputs=+
  Out1 : Outport
  wires:
  Sum of Elements1/1 -> Sqrt/1
  Math Function2/1 -> Sum of Elements1/1
  Sqrt/1 -> Out1/1
  In1/1 -> Math Function2/1

== system Marine_LocoMotive_UAV/Preprocessing Unit/Alpha_bar/smooth switch ==
  u 1 : Inport
  u 2 : Inport  Port=2
  switch : Inport  Port=3
  Constant : Constant
  Data Type Conversion : DataTypeConversion
  Low Pass Filter2 : DiscreteTransferFcn  Numerator=Bm_asw_LPF  Denominator=Am_asw_LPF
  Product : Product
  Product1 : Product
  Step1 : Step  SampleTime=0
  Subtract : Sum  Inputs=+-
  Sum : Sum  Inputs=|++
  "switch " : Scope
  y : Outport
  wires:
  Product/1 -> Sum/2
  Product1/1 -> Sum/1
  Low Pass Filter2/1 -> "switch "/1, Product/1, Subtract/2
  Data Type Conversion/1 -> Low Pass Filter2/1
  u 1/1 -> Product1/1
  u 2/1 -> Product/2
  switch/1 -> Data Type Conversion/1
  Sum/1 -> y/1
  Constant/1 -> Subtract/1
  Subtract/1 -> Product1/2

== system Marine_LocoMotive_UAV/Preprocessing Unit/T_bar /Damping coefficient estimation ==
  note: Friction damping coeficients estimation
  C_s_bar : Scope
  "D11 " : Scope
  "D11_0 " : Scope
  Delay : Delay  DelayLength=1  InitialCondition=0
  Vol_im_bar to Dh_bar : Subsystem
  advanced damping estimates : Subsystem
  damping estimates : Subsystem
  "mean skin friction coefficient " : Subsystem
  D11_0 : Outport
  D11_bar : Outport  Port=2
  wires:
  Delay/1 -> D11_bar/1, "D11 "/1
  [V_bar] -> "mean skin friction coefficient "/1(V)
  [V_r_bar] -> advanced damping estimates/1(Vr_bar)
  advanced damping estimates/1(D11) -> Delay/1
  Vol_im_bar to Dh_bar/1(D) -> advanced damping estimates/2(Dh_bar)
  damping estimates/1(D11,0) -> D11_0/1, "D11_0 "/1
  "mean skin friction coefficient "/1(C_S) -> C_s_bar/1, [C_S_bar]
  [Vol_im_bar] -> Vol_im_bar to Dh_bar/1(V)
  [V_bar] -> damping estimates/1(V_bar)
  [C_S_bar] -> damping estimates/2(C_S_bar)
  [C_S_bar] -> advanced damping estimates/3(C_S)

== system Marine_LocoMotive_UAV/Preprocessing Unit/T_bar /Tension from UAV, X and r directions ==
  alpha : Inport
  theta_u : Inport  Port=2
  u1 : Inport  Port=3
  Xu_ddot : Inport  Port=4
  Add3 : Sum  Inputs=+--
  Constant : Constant  Value=m_u*g
  Gain14 : Gain
  Gain15 : Gain  Gain=m_u
  Product12 : Product
  Product9 : Product  Inputs=*/
  Trigonometric Function6 : Trigonometry
  Trigonometric Function8 : Trigonometry  Operator=cos
  x_ddot1 : Selector  InputPortWidth=2  IndexOptions=Index vector (dialog)  Indices=2  OutputSizes=1
  "T, from x simple" : Outport
  wires:
  Product9/1 -> "T, from x simple"/1
  Add3/1 -> Product9/1
  Gain14/1 -> Add3/1
  Trigonometric Function8/1 -> Product12/1
  u1/1 -> Product12/2
  alpha/1 -> Trigonometric Function6/1
  Product12/1 -> Gain14/1
  x_ddot1/1 -> Gain15/1
  Trigonometric Function6/1 -> Product9/2
  Xu_ddot/1 -> x_ddot1/1
  theta_u/1 -> Trigonometric Function8/1
  Gain15/1 -> Add3/2
  Constant/1 -> Add3/3

== system Marine_LocoMotive_UAV/Preprocessing Unit/T_bar /skip near pi//2 region ==
  In1 : Inport
  Constant : Constant  Value=80*pi/180
  Constant2 : Constant  Value=100*pi/180
  MinMax : MinMax
  MinMax1 : MinMax  Function=max
  Switch : Switch  Criteria=u2 > Threshold  Threshold=pi/2
  Vector Concatenate6 : Concatenate
  Vector Concatenate7 : Concatenate
  Out1 : Outport
  wires:
  Vector Concatenate7/1 -> MinMax1/1
  MinMax/1 -> Switch/3
  In1/1 -> Vector Concatenate6/1, Switch/2, Vector Concatenate7/2
  Vector Concatenate6/1 -> MinMax/1
  Constant2/1 -> Vector Concatenate7/1
  MinMax1/1 -> Switch/1
  Constant/1 -> Vector Concatenate6/2
  Switch/1 -> Out1/1

== system Marine_LocoMotive_UAV/Preprocessing Unit/T_bar /skip near pi//2 region1 ==
  In1 : Inport
  Constant : Constant  Value=80*pi/180
  Constant2 : Constant  Value=100*pi/180
  MinMax : MinMax
  MinMax1 : MinMax  Function=max
  Switch : Switch  Criteria=u2 > Threshold  Threshold=pi/2
  Vector Concatenate6 : Concatenate
  Vector Concatenate7 : Concatenate
  Out1 : Outport
  wires:
  Vector Concatenate7/1 -> MinMax1/1
  MinMax/1 -> Switch/3
  In1/1 -> Vector Concatenate6/1, Switch/2, Vector Concatenate7/2
  Vector Concatenate6/1 -> MinMax/1
  Constant2/1 -> Vector Concatenate7/1
  MinMax1/1 -> Switch/1
  Constant/1 -> Vector Concatenate6/2
  Switch/1 -> Out1/1

== system Marine_LocoMotive_UAV/Preprocessing Unit/T_bar /smooth lower bound ==
  u : Inport
  Manual Switch : ManualSwitch
  Mux3 : Mux  Inputs=2
  Saturation1 : Saturate  UpperLimit=inf  LowerLimit=min_sf
  apply for lower bound only : Switch  Criteria=u2 > Threshold  Threshold=Amp_sf+min_sf
  sat : Scope
  saturation function : Fcn  Expr=Amp_sf*tanh((u(1)-(Amp_sf+min_sf))/(Amp_sf)) + (Amp_sf+min_sf)
  sat(u) : Outport
  wires:
  Manual Switch/1 -> sat(u)/1
  Saturation1/1 -> Manual Switch/2
  u/1 -> saturation function/1, apply for lower bound only/2, Mux3/1, apply for lower bound only/1, Saturation1/1
  saturation function/1 -> apply for lower bound only/3, Mux3/2
  Mux3/1 -> sat/1
  apply for lower bound only/1 -> Manual Switch/1

== system Marine_LocoMotive_UAV/Preprocessing Unit/T_bar /smooth lower bound1 ==
  u : Inport
  Manual Switch : ManualSwitch
  Mux3 : Mux  Inputs=2
  Saturation1 : Saturate  UpperLimit=inf  LowerLimit=min_sf
  apply for lower bound only : Switch  Criteria=u2 > Threshold  Threshold=Amp_sf+min_sf
  sat : Scope
  saturation function : Fcn  Expr=Amp_sf*tanh((u(1)-(Amp_sf+min_sf))/(Amp_sf)) + (Amp_sf+min_sf)
  sat(u) : Outport
  wires:
  apply for lower bound only/1 -> Manual Switch/1
  Mux3/1 -> sat/1
  saturation function/1 -> Mux3/2, apply for lower bound only/3
  u/1 -> Saturation1/1, apply for lower bound only/1, Mux3/1, apply for lower bound only/2, saturation function/1
  Saturation1/1 -> Manual Switch/2
  Manual Switch/1 -> sat(u)/1

== system Marine_LocoMotive_UAV/Quadrotor+buoy/3-DOF equations of motion Earth frame/C_123 ==
  "alpha " : Inport
  alpha_dot : Inport  Port=2
  coupled : Inport  Port=3
  Constant : Constant  Value=0
  Constant1 : Constant  Value=m_u
  Gain : Gain  Gain=-L
  Gain1 : Gain  Gain=-L
  Product : Product  Inputs=3
  Product1 : Product  Inputs=3
  Product2 : Product
  Signal Specification1 : SignalSpecification  Dimensions=3
  Signal Specification2 : SignalSpecification  Dimensions=3
  Signal Specification3 : SignalSpecification  Dimensions=3
  Trigonometric Function : Trigonometry  Operator=sincos
  Vector Concatenate1 : Concatenate  NumInputs=3  Mode=Multidimensional array  ConcatenateDimension=2
  Vector Concatenate2 : Concatenate  NumInputs=3
  Vector Concatenate3 : Concatenate  NumInputs=3
  Vector Concatenate4 : Concatenate  NumInputs=3
  C_123 : Outport
  wires:
  Signal Specification3/1 -> Vector Concatenate1/3
  Signal Specification2/1 -> Vector Concatenate1/2
  Signal Specification1/1 -> Vector Concatenate1/1
  Vector Concatenate1/1 -> C_123/1
  Trigonometric Function/2 -> Gain1/1
  Trigonometric Function/1 -> Gain/1
  "alpha "/1 -> Trigonometric Function/1
  Vector Concatenate4/1 -> Signal Specification2/1
  Vector Concatenate2/1 -> Signal Specification1/1
  Vector Concatenate3/1 -> Signal Specification3/1
  Gain/1 -> Product/2
  Gain1/1 -> Product1/2
  Product1/1 -> Vector Concatenate3/1
  Product/1 -> Vector Concatenate3/2
  alpha_dot/1 -> Product1/3, Product/3
  Constant/1 -> Vector Concatenate3/3, Vector Concatenate4/3, Vector Concatenate4/2, Vector Concatenate4/1, Vector Concatenate2/3, Vector Concatenate2/2, Vector Concatenate2/1
  coupled/1 -> Product2/1
  Constant1/1 -> Product2/2
  Product2/1 -> Product1/1, Product/1

== system Marine_LocoMotive_UAV/Quadrotor+buoy/3-DOF equations of motion Earth frame/Coupling state ==
  pos_T : Inport
  re_couple : Inport  Port=2
  Data Type Conversion : DataTypeConversion  OutDataTypeStr=double
  Delay10 : Delay  DelayLength=1  InitialCondition=1
  IC3 : InitialCondition
  IC5 : InitialCondition  Value=coupled_ini
  MATLAB Function : MATLAB Function  TreatAsAtomicUnit=on
  "T, r,xu,xb1" : Scope
  break algebraic loop : Delay  DelayLength=1  InitialCondition=1
  "is coupled " : Scope
  is coupled -1 : Scope
  pos tension : Scope
  positive tension : Scope
  "positive tension with gap " : simulink/Logic and Bit Operations/Compare To Constant  relop=>  const=0-0.01  OutDataTypeStr=boolean
  "re_couple " : Scope
  state detector : Scope
  is coupled : Outport
  wires:
  Delay10/1 -> is coupled -1/1, MATLAB Function/3(coupled)
  IC5/1 -> is coupled/1, Delay10/1
  MATLAB Function/1(is_coupled) -> IC5/1, "is coupled "/1
  break algebraic loop/1 -> pos tension/1, MATLAB Function/1(pos_T)
  re_couple/1 -> MATLAB Function/2(re_couple), "re_couple "/1
  MATLAB Function/2(c) -> state detector/1
  pos_T/1 -> "T, r,xu,xb1"/1, "positive tension with gap "/1
  Data Type Conversion/1 -> positive tension/1, break algebraic loop/1
  IC3/1 -> Data Type Conversion/1
  "positive tension with gap "/1 -> IC3/1

== system Marine_LocoMotive_UAV/Quadrotor+buoy/3-DOF equations of motion Earth frame/D_123 ==
  eta_dot_tilde : Inport
  theta_b : Inport  Port=2
  dh : Inport  Port=3
  Constant6 : Constant  Value=[0 0 0]
  Constant7 : Constant  Value=0
  Scope : Scope
  Scope1 : Scope
  Scope2 : Scope
  Signal Specification2 : SignalSpecification  Dimensions=[3 3]
  Vector Concatenate1 : Concatenate  NumInputs=3  Mode=Multidimensional array  ConcatenateDimension=2
  Vector Concatenate2 : Concatenate  NumInputs=3
  Vector Concatenate3 : Concatenate  NumInputs=3
  Vector Concatenate4 : Concatenate
  Vector Concatenate5 : Concatenate
  Vector Concatenate6 : Concatenate
  Water Daming : Subsystem
  Water Daming1 : Subsystem
  D_123 : Outport
  wires:
  Water Daming/2(D22_I) -> Vector Concatenate3/2, Vector Concatenate5/2
  Constant7/1 -> Vector Concatenate3/3, Vector Concatenate2/3
  Constant6/1 -> Vector Concatenate1/3
  Vector Concatenate2/1 -> Vector Concatenate1/1
  Water Daming/1(D11_I) -> Vector Concatenate4/2, Vector Concatenate2/1
  Vector Concatenate3/1 -> Vector Concatenate1/2
  theta_b/1 -> Water Daming1/1(theta), Water Daming/1(theta_b)
  eta_dot_tilde/1 -> Water Daming/2(eta_dot_tilde)
  dh/1 -> Water Daming/3(dh)
  Vector Concatenate1/1 -> Signal Specification2/1
  Vector Concatenate4/1 -> Scope/1
  Water Daming1/1(D11_I) -> Vector Concatenate4/1
  Vector Concatenate5/1 -> Scope1/1
  Water Daming1/2(D22_I) -> Vector Concatenate5/1
  Vector Concatenate6/1 -> Scope2/1
  Water Daming1/3(D12_I) -> Vector Concatenate6/1
  Water Daming/3(D12_I) -> Vector Concatenate3/1, Vector Concatenate6/2, Vector Concatenate2/2
  Signal Specification2/1 -> D_123/1

== system Marine_LocoMotive_UAV/Quadrotor+buoy/3-DOF equations of motion Earth frame/D_u (vector for simplification) ==
  Vr : Inport
  A.Q.Cd : Product
  Abs : Abs
  Cd x A : Constant  Value=Cd_u*Ac
  rho/2 : Gain  Gain=rho_a/2
  Du : Outport
  wires:
  Vr/1 -> Abs/1
  Cd x A/1 -> A.Q.Cd/2
  rho/2/1 -> A.Q.Cd/1
  Abs/1 -> rho/2/1
  A.Q.Cd/1 -> Du/1

== system Marine_LocoMotive_UAV/Quadrotor+buoy/3-DOF equations of motion Earth frame/FB ==
  Constant1 : Constant  Value=rho_w*g
  F_B : Product
  Out1 : Outport
  wires:
  F_B/1 -> Out1/1
  [Vol_im] -> F_B/1
  Constant1/1 -> F_B/2

== system Marine_LocoMotive_UAV/Quadrotor+buoy/3-DOF equations of motion Earth frame/G1 ==
  Constant3 : Constant  Value=0
  Constant4 : Constant  Value=(m_b)*g
  Vector Concatenate : Concatenate
  G : Outport
  wires:
  Vector Concatenate/1 -> G/1
  Constant3/1 -> Vector Concatenate/1  "u1"
  Constant4/1 -> Vector Concatenate/2  "u2"

== system Marine_LocoMotive_UAV/Quadrotor+buoy/3-DOF equations of motion Earth frame/G123 ==
  alpha : Inport
  coupled : Inport  Port=2
  Constant : Constant  Value=m_b
  Constant3 : Constant  Value=0
  Constant4 : Constant  Value=m_u
  Constant5 : Constant  Value=g*L
  Gain1 : Gain  Gain=g
  Product : Product
  Product5 : Product  Inputs=3  SaturateOnIntegerOverflow=on  InputSameDT=on  OutDataTypeStr=Inherit: Same as first input
  Sum : Sum  Inputs=|++
  Trigonometric Function : Trigonometry  Operator=cos
  Vector Concatenate : Concatenate  NumInputs=3
  G : Outport
  wires:
  Constant5/1 -> Product5/1
  Trigonometric Function/1 -> Product5/2
  Product5/1 -> Vector Concatenate/3  "u3"
  Gain1/1 -> Vector Concatenate/2  "u2"
  Constant3/1 -> Vector Concatenate/1  "u1"
  alpha/1 -> Trigonometric Function/1
  Vector Concatenate/1 -> G/1
  Constant/1 -> Sum/2
  coupled/1 -> Product/1
  Constant4/1 -> Product/2  "u2"
  Sum/1 -> Gain1/1
  Product/1 -> Product5/3, Sum/1
